simulink model "shiyufx"  (Simulink 3.00)
settings: Solver=ode45  StartTime=0.0  StopTime=20  RelTol=1e-3

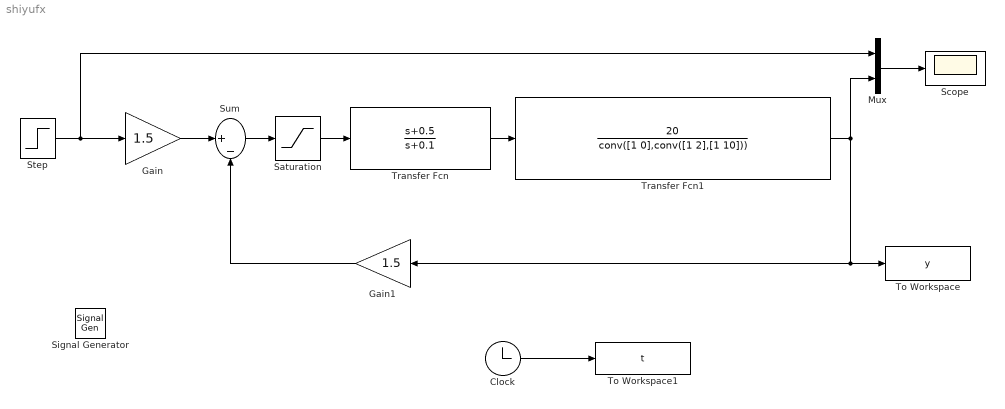
== system shiyufx ==
  Clock : Clock
      settings: DisplayTime=off  Decimation=10
  Gain : Gain  Gain=1.5  SaturateOnIntegerOverflow=on
  Gain1 : Gain  Orientation=left  Gain=1.5  SaturateOnIntegerOverflow=on
  Mux : Mux  Inputs=2
  Saturation : Saturate  UpperLimit=0.5  LowerLimit=-0.2
  Scope : Scope
      settings: TimeRange=20  YMin=-1.4  YMax=1.5  SaveToWorkspace=off  SaveName=ScopeData  LimitMaxRows=off
  Signal Generator : SignalGenerator  WaveForm=sine  Amplitude=1  Frequency=1  Units=Hertz
  Step : Step  Time=1  Before=0  After=1  SampleTime=0
  Sum : Sum  Inputs=|+-  SaturateOnIntegerOverflow=on
  To Workspace : ToWorkspace  VariableName=y  SampleTime=-1  SaveFormat=Matrix
  To Workspace1 : ToWorkspace  VariableName=t  SampleTime=-1  SaveFormat=Matrix
  Transfer Fcn : TransferFcn  Numerator=[1 0.5]  Denominator=[1 0.1]
  Transfer Fcn1 : TransferFcn  Numerator=[20]  Denominator=conv([1 0],conv([1 2],[1 10]))
  wires:
  Gain/1 -> Sum/1
  Transfer Fcn/1 -> Transfer Fcn1/1
  Gain1/1 -> Sum/2
  Clock/1 -> To Workspace1/1
  Step/1 -> Gain/1, Mux/1
  Sum/1 -> Saturation/1
  Saturation/1 -> Transfer Fcn/1
  Mux/1 -> Scope/1
  Transfer Fcn1/1 -> Gain1/1, To Workspace/1, Mux/2
